simulink model "ControlTopH11"  (R2026a)
settings: Solver=FixedStepDiscrete  StopTime=Inf  FixedStep=0.0005  EnableMultiTasking=on
undefined symbols (not defined in the file or in its folder): P_in, P_out
settings Model: Creator=Mutti  LastModifiedBy=Mutti
settings DataIOCC: SaveState=on  InspectSignalLogs=on
settings OptimizationCC: StrengthReduction=on  MaxStackSize=512  OptimizationPriority=Speed  UseRestrictQualifier=on
settings HardwareCC: ProdLargestAtomicInteger=Long  ProdLargestAtomicFloat=Double  ProdHWDeviceType=ARM Compatible->ARM Cortex-M
settings ModelReferenceCC: PropagateVarSize=During execution
settings RTWCC: SystemTargetFile=ert.tlc  GenCodeOnly=on  GenerateReport=on  BuildConfiguration=Faster Runs  IncludeHyperlinkInReport=on  LaunchReport=on  PortableWordSizes=on  CodeProfilingSaveOptions=AllData  TargetLang=C++  GenerateTraceInfo=on  GenerateTraceReport=on  GenerateTraceReportSl=on  GenerateTraceReportSf=on  GenerateTraceReportEml=on  GenerateWebview=on  GenerateCodeMetricsReport=on  GenerateCodeReplacementReport=on  Description=Embedded Coder
settings CodeAppCC: GenerateComments=off  SimulinkBlockComments=off
settings ERTTargetCC: ExtModeTransport=3.0  ExtModeStaticAllocSize=2048.0  RootIOFormat=Structure reference  TargetLangStandard=C++20 (ISO)  CodeReplacementLibrary=ARM Cortex-M  CodeInterfacePackaging=C++ class  SubcomponentCodeInterfacePackaging=C++ class  SupportNonFinite=off  SupportVariableSizeSignals=on

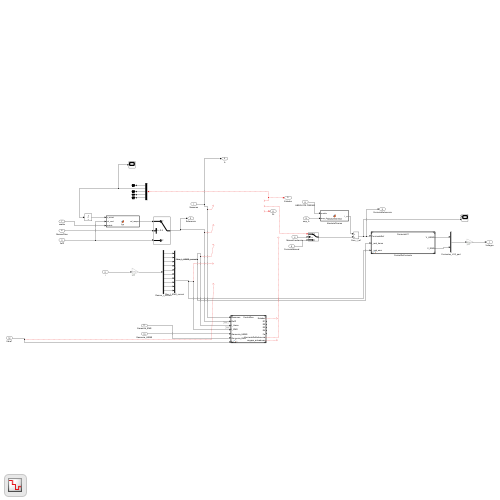
[thumbnail: Simulink's stored preview of the top-level diagram]
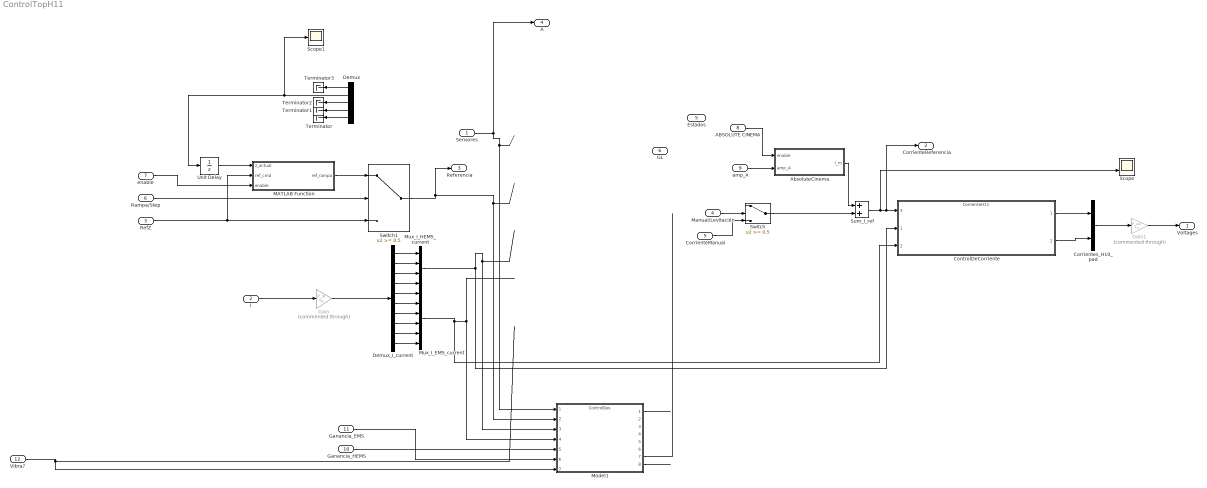
== system ControlTopH11 ==
  Sensores : Inport
  I : Inport  Port=2
  RefZ : Inport  Port=3
  Manual/Levitación : Inport  Port=4
  CorrienteManual : Inport  Port=5  PortDimensions=10
  Rampa/Step : Inport  Port=6
  enable : Inport  Port=7
  ABSOLUTE CINEMA : Inport  Port=8
  amp_A : Inport  Port=9
  Ganancia_HEMS : Inport  Port=10  OutDataTypeStr=uint8
  Ganancia_EMS : Inport  Port=11  OutDataTypeStr=uint8
  Vibra? : Inport  Port=12  OutDataTypeStr=boolean
  AbsoluteCInema : MATLAB Function  TreatAsAtomicUnit=on
  ControlDeCorriente : ModelReference  ModelNameDialog=CorrienteH11.slx  SimulationMode=Normal  ModelReferenceVersion=2.34
      settings: PortSchema="{\"entries\":[{\"content\":{\"sides\":[{\"content\":{\"connectorIds\":[\"In3\",\"In1\",\"In2\"]},\"type\":\"ConnectorPlacement.EquallySpacedRectSide\",\"uuid\":\"5729e6b8-d772-49de-a6ae-f4854e6c636c\"},{\"content\":{\"connectorIds\":[\"Out1\",\"Out2\"],\"side\":\"RIGHT\"},\"type\":\"ConnectorPlacement.EquallySpacedRectSide\",\"uuid\":\"5b4533a2-f460-4d30-aa00-3ce7774336b6\"},{\"content\":{\"side\":\"TOP\"},\"type\":\"ConnectorPlacement.EquallySpacedRectSide\",\"uuid\":\"49b747cd-7600-4dea-82cc-ca0520f6a6ff\"}]},\"type\":\"ConnectorPlacement.EquallySpacedConnector\",\"uuid\":\"73e3d239-930b-41eb-a7f4-eb5adfeb43ac\"}],\"packageUris\":[\"http://schema.mathworks.com/mf0/Connector/R2020b\"],\"version\":\"1.0\"}"
  Corrientes_H10_pad : Mux  Inputs=2
  Demux : Demux  Outputs=5
  Demux_I_current : Demux  Outputs=10
  Gain : Gain  Commented=through  Gain=P_in  Multiplication=Matrix(K*u)
  Gain1 : Gain  Commented=through  Gain=P_out  Multiplication=Matrix(K*u)
  MATLAB Function : MATLAB Function  TreatAsAtomicUnit=on
  Model1 : ModelReference  ModelNameDialog=ControlDes.slx  SimulationMode=Normal  ModelReferenceVersion=8.121
  Mux_I_EMS_current : Mux  Inputs=6
  Mux_I_HEMS_current : Mux
  Scope : Scope  NumInputPorts=2
      settings: ActiveDisplayYMinimum=-437.5  ActiveDisplayYMaximum=437.5
  Scope1 : Scope
      settings: ActiveDisplayYMinimum=-1  ActiveDisplayYMaximum=1
  Sum_I_ref : Sum  OutDataTypeStr=double
  Switch : Switch  Threshold=0.5  SaturateOnIntegerOverflow=off  InputSameDT=off
  Switch1 : Switch  Threshold=0.5  SaturateOnIntegerOverflow=off  InputSameDT=off
  Terminator{,1..3} (4 alike) : Terminator
  Unit Delay : UnitDelay  SampleTime=-1
  Voltages : Outport
  CorrienteReferencia : Outport  Port=2
  Referencia : Outport  Port=3
  A : Outport  Port=4
  Estados : Outport  Port=5
  GL : Outport  Port=6
  wires:
  Sensores/1 -> A/1, Model1/1
  Manual/Levitación/1 -> Switch/2
  ControlDeCorriente/1 -> Corrientes_H10_pad/1
  Switch/1 -> Sum_I_ref/2
  CorrienteManual/1 -> Switch/3
  RefZ/1 -> MATLAB Function/2(ref_cmd), Switch1/3
  MATLAB Function/1(ref_rampa) -> Switch1/1
  Switch1/1 -> Referencia/1, Model1/2
  Rampa/Step/1 -> Switch1/2
  Unit Delay/1 -> MATLAB Function/1(z_actual)
  Demux/2 -> Scope1/1, Unit Delay/1
  Demux/5 -> Terminator/1
  Demux/4 -> Terminator1/1
  Demux/3 -> Terminator2/1
  Demux/1 -> Terminator3/1
  enable/1 -> MATLAB Function/3(enable)
  ? -> Demux/1, Estados/1
  ABSOLUTE CINEMA/1 -> AbsoluteCInema/1(enable)
  amp_A/1 -> AbsoluteCInema/2(amp_A)
  AbsoluteCInema/1(I_m) -> Sum_I_ref/1
  ControlDeCorriente/2 -> Corrientes_H10_pad/2
  Sum_I_ref/1 -> CorrienteReferencia/1, ControlDeCorriente/3, Scope/2
  I/1 -> Gain/1
  Demux_I_current/1 -> Mux_I_HEMS_current/1
  Demux_I_current/2 -> Mux_I_HEMS_current/2
  Demux_I_current/3 -> Mux_I_HEMS_current/3
  Demux_I_current/4 -> Mux_I_HEMS_current/4
  Demux_I_current/5 -> Mux_I_EMS_current/1
  Demux_I_current/6 -> Mux_I_EMS_current/2
  Demux_I_current/7 -> Mux_I_EMS_current/3
  Demux_I_current/8 -> Mux_I_EMS_current/4
  Demux_I_current/9 -> Mux_I_EMS_current/5
  Demux_I_current/10 -> Mux_I_EMS_current/6
  Mux_I_EMS_current/1 -> Model1/4, ControlDeCorriente/2
  Mux_I_HEMS_current/1 -> ControlDeCorriente/1, Model1/3
  Gain/1 -> Demux_I_current/1
  Corrientes_H10_pad/1 -> Gain1/1
  Gain1/1 -> Voltages/1
  Model1/1 -> ?
  Model1/8 -> ?
  ? -> Switch/1
  Model1/7 -> ?
  Ganancia_HEMS/1 -> Model1/5
  Ganancia_EMS/1 -> Model1/6
  Vibra?/1 -> Model1/7
  ? -> GL/1

== matlab function ControlTopH11/AbsoluteCInema ==
  data: enable input; I_m output; amp_A input
function I_m = AbsoluteCinema(enable, amp_A)
%#codegen
% Recursive oscillator music current injector for four HEMS and six EMS coils.
% The HEMS pattern is [+a; -a; -a; +a]; EMS channels use positive abs(a).

persistent note_idx sample_in_note s c freqs durs gains sinInc cosInc

Ts = 1.0 / 2000.0;
attack_samples = uint32(20);  % 10 ms at 2 kHz.
release_samples = uint32(20); % 10 ms at 2 kHz.

I_m = zeros(10, 1);

if isempty(note_idx)
    [freqs_s, durs_s, gains_s, sinInc_s, cosInc_s] = music_injector_data();
    freqs = double(freqs_s);
    durs = double(durs_s);
    gains = double(gains_s);
    sinInc = double(sinInc_s);
    cosInc = double(cosInc_s);
    note_idx = uint32(1);
    sample_in_note = uint32(0);
    s = 0.0;
    c = 1.0;
end

if enable == 0
    note_idx = uint32(1);
    sample_in_note = uint32(0);
    s = 0.0;
    c = 1.0;
    return;
end

note_count = uint32(numel(freqs));
if note_count == 0
    return;
end

if note_idx > note_count
    note_idx = uint32(1);
    sample_in_note = uint32(0);
    s = 0.0;
    c = 1.0;
end

note_samples_f = durs(note_idx) / Ts;
note_samples = uint32(max(1.0, floor(note_samples_f + 0.5)));

env = 1.0;
if sample_in_note < attack_samples
    env = min(env, double(sample_in_note) / double(attack_samples));
end

samples_left = note_samples - min(sample_in_note, note_samples);
if samples_left < release_samples
    env = min(env, double(samples_left) / double(release_samples));
end

amp = double(amp_A);
if amp < 0.0
    amp = 0.0;
end

a = amp * gains(note_idx) * env * s;
I_m(1) = a;
I_m(2) = -a;
I_m(3) = -a;
I_m(4) = a;

a_ems = abs(a);
I_m(5) = a_ems;
I_m(6) = a_ems;
I_m(7) = a_ems;
I_m(8) = a_ems;
I_m(9) = a_ems;
I_m(10) = a_ems;

s_delta = sinInc(note_idx);
c_delta = cosInc(note_idx);
s_next = s * c_delta + c * s_delta;
c_next = c * c_delta - s * s_delta;
s = s_next;
c = c_next;

sample_in_note = sample_in_note + uint32(1);
if sample_in_note >= note_samples
    sample_in_note = uint32(0);
    note_idx = note_idx + uint32(1);
    if note_idx > note_count
        note_idx = uint32(1);
    end
    s = 0.0;
    c = 1.0;
end

end

== matlab function ControlTopH11/MATLAB Function ==
  data: z_actual input; ref_rampa output; ref_cmd input; enable input
function ref_rampa = fcn(z_actual, ref_cmd, enable)
% Rampa de referencia robusta para MCU
% Unidades: metros

Ts = 0.001;          % [s]
v  = 0.005;          % [m/s] = 3 mm/s
step = v * Ts;       % [m] = 3e-6 m por muestra

persistent ref

% 1. Inicialización segura
if isempty(ref)
    ref = z_actual;
end

% 2. Máquina de estados simplificada
if enable == 0
    % Mientras NO esté activa, la rampa persigue continuamente la posición real.
    % Así, en el momento exacto en que 'enable' pase a 1, 'ref' ya contendrá
    % los 25mm exactos, listos para empezar a iterar.
    ref = z_actual;
else
    % Modo Rampa: Una vez activo, persigue a ref_cmd paso a paso
    e = ref_cmd - ref;

    if e > step
        ref = ref + step;
    elseif e < -step
        ref = ref - step;
    else
        ref = ref_cmd;
    end
end

ref_rampa = ref;
